simulink model "example_frequency_response"  (R2021b)
settings: Solver=FixedStepDiscrete  StartTime=0.0  StopTime=min(2*3600,15/quadruple_example_frequency_response_f)  FixedStep=0.5  RelTol=1e-3
undefined symbols (not defined in the file or in its folder): cte, quadruple_example_frequency_response_A, quadruple_example_frequency_response_Ai, quadruple_example_frequency_response_f
libraries: sldrtlib x1, simulink x1
settings Model: Creator=IST  LastModifiedBy=IST

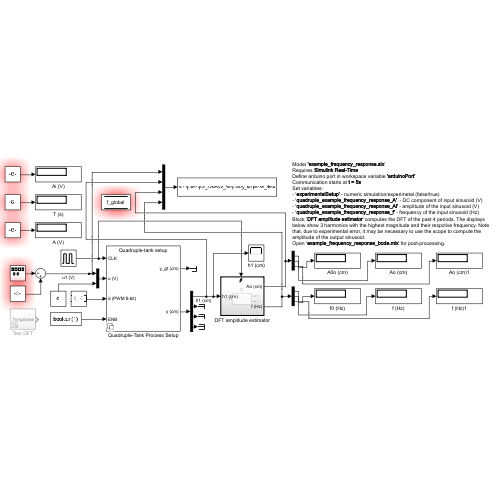
[thumbnail: Simulink's stored preview of the top-level diagram]
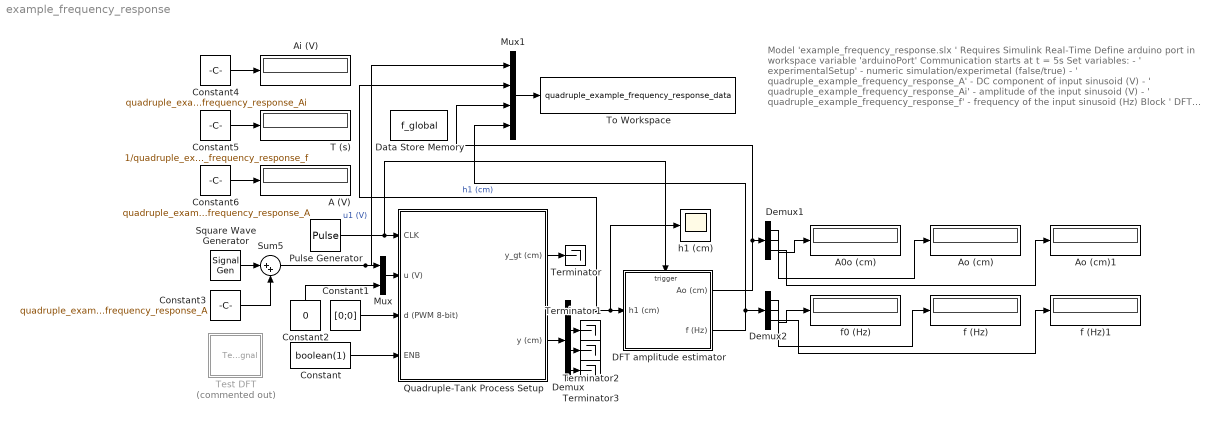
== system example_frequency_response ==
  note: Model 'example_frequency_response.slx '
      | Requires Simulink Real-Time
      | Define arduino port in workspace variable 'arduinoPort'
      | Communication starts at t = 5s
      | Set variables:
      | - ' experimentalSetup' - numeric simulation/experimetal (false/true)
      | - ' quadruple_example_frequency_response_A' - DC component of input sinusoid (V)
      | - ' quadruple_example_frequency_response_Ai' - amplitude of the input sinusoid (V)
      | - ' quadruple_example_frequency_response_f' - frequency of the input sinusoid (Hz)
      | Block ' DFT amplitude estimator ' computes the DFT of the past 4 periods. The displays below show 3 harmonics with the highest magnitude and their respctive frequency. Note that, due to experimental error, it may be necessary to use the scope to compute the amplitude of the output sinusoid.
      | Open ' example_frequency_response_bode.mlx ' for post-processing.
  A (V) : Display
  A0o (cm) : Display
  Ai (V) : Display
  Ao (cm) : Display
  Ao (cm)1 : Display
  Constant : Constant  Priority=4  Value=boolean(1)
  Constant1 : Constant  Value=[0;0]
  Constant2 : Constant  Value=0
  Constant3 : Constant  Value=quadruple_example_frequency_response_A
  Constant4 : Constant  Value=quadruple_example_frequency_response_Ai
  Constant5 : Constant  Value=1/quadruple_example_frequency_response_f
  Constant6 : Constant  Value=quadruple_example_frequency_response_A
  DFT amplitude estimator : Subsystem
  Data Store Memory : DataStoreMemory  DataStoreName=f_global  ReadBeforeWriteMsg=warning  WriteAfterWriteMsg=warning  WriteAfterReadMsg=warning  InitialValue=quadruple_example_frequency_response_f  ShowAdditionalParam=off  OutDataTypeStr=double
  Demux : Demux
  Demux1 : Demux  Outputs=3
  Demux2 : Demux  Outputs=3
  Mux : Mux  Inputs=2
  Mux1 : Mux
  Pulse Generator : DiscretePulseGenerator  PulseType=Time based  Period=1  PulseWidth=50
  Quadruple-Tank Process Setup : Subsystem  InitFcn=|  StopFcn=|  Variant=on
      InitFcn=|
      | % Load parameters
      | cte = quadrupleLoadParameters();
      | % Select simulation mode if unspecified
      | if ~exist('experimentalSetup')
      | experimentalSetup = false;
      | end
      | if experimentalSetup
      | if exist('arduinoPort')
      | if ~isempty(instrfind)
      | fclose(instrfind);
      | delete(instrfind);
      | end
      | arduino = serial(arduinoPort,...
      |                 'BaudRate',9600,...
      |                 'ByteOrder','bigEndian',...
      |                 'DataBits',8,...
      |                 'StopBits',1,...
      |                 'Terminator','');
      | arduino.Parity = 'none';
      | fopen(arduino);
      | else
      | error("Error: Arduino port undefined. Define the port in workspace variable 'arduinoPort'.");
      | end
      | end
      StopFcn=|
      | if experimentalSetup
      | fclose(arduino);
      | end
  Square Wave Generator : SignalGenerator  Amplitude=quadruple_example_frequency_response_Ai  Frequency=quadruple_example_frequency_response_f
  Sum5 : Sum  Inputs=|++
  T (s) : Display
  Terminator{,1..3} (4 alike) : Terminator
  Test DFT : Subsystem  Commented=on
  To Workspace : ToWorkspace  VariableName=quadruple_example_frequency_response_data  SaveFormat=Timeseries  SampleTime=1
  f (Hz) : Display
  f (Hz)1 : Display
  f0 (Hz) : Display
  h1 (cm) : Scope
  wires:
  Demux1/3 -> Ao (cm)1/1
  Demux1/2 -> Ao (cm)/1
  Demux2/3 -> f (Hz)1/1
  Demux/2 -> Terminator1/1
  Constant5/1 -> T (s)/1
  Demux2/2 -> f (Hz)/1
  DFT amplitude estimator/2(f (Hz)) -> Mux1/4, Demux2/1
  Mux/1 -> Quadruple-Tank Process Setup/2(u (V))
  Demux1/1 -> A0o (cm)/1
  Pulse Generator/1 -> Quadruple-Tank Process Setup/1(CLK), DFT amplitude estimator/Trigger
  Constant6/1 -> A (V)/1
  Constant1/1 -> Quadruple-Tank Process Setup/3(d (PWM 8-bit))
  Constant4/1 -> Ai (V)/1
  Mux1/1 -> To Workspace/1
  Demux2/1 -> f0 (Hz)/1
  DFT amplitude estimator/1(Ao (cm)) -> Demux1/1, Mux1/3
  Square Wave Generator/1 -> Sum5/1
  Sum5/1 -> Mux1/1, Mux/1  "u1 (V)"
  Demux/1 -> Mux1/2, h1 (cm)/1, DFT amplitude estimator/1(h1 (cm))  "h1 (cm)"
  Quadruple-Tank Process Setup/1(y_gt (cm)) -> Terminator/1
  Constant3/1 -> Sum5/2
  Quadruple-Tank Process Setup/2(y (cm)) -> Demux/1
  Constant2/1 -> Mux/2
  Demux/3 -> Terminator2/1
  Demux/4 -> Terminator3/1
  Constant/1 -> Quadruple-Tank Process Setup/4(ENB)

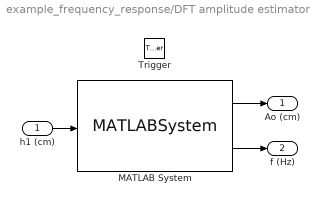
== system example_frequency_response/DFT amplitude estimator ==
  h1 (cm) : Inport
  Trigger : TriggerPort  VariantControl=Variant  PortDimensions=1
  MATLAB System : MATLABSystem  System=output_amplitude_dft  SimulateUsing=Code generation
      mask Type: output_amplitude_dft
      mask Display:
      | disp('output_amplitude_dft');
      | port_label('input',1,'y');
      | port_label('output',1,'Ao');
      | port_label('output',2,'f');
  Ao (cm) : Outport  VectorParamsAs1DForOutWhenUnconnected=off
  f (Hz) : Outport  Port=2  VectorParamsAs1DForOutWhenUnconnected=off
  wires:
  MATLAB System/1 -> Ao (cm)/1
  h1 (cm)/1 -> MATLAB System/1
  MATLAB System/2 -> f (Hz)/1

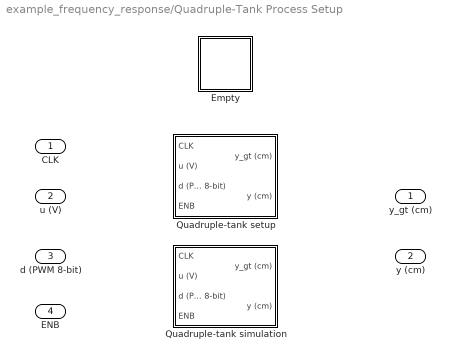
== system example_frequency_response/Quadruple-Tank Process Setup ==
  CLK : Inport
  u (V) : Inport  Port=2
  d (PWM 8-bit) : Inport  Port=3
  ENB : Inport  Port=4
  Empty : Subsystem  VariantControl=%
  Quadruple-tank setup : Subsystem  VariantControl=experimentalSetup == true
  Quadruple-tank simulation : Subsystem  Priority=4  VariantControl=experimentalSetup == false
  y_gt (cm) : Outport  VectorParamsAs1DForOutWhenUnconnected=off
  y (cm) : Outport  Port=2  VectorParamsAs1DForOutWhenUnconnected=off

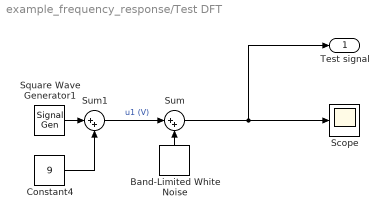
== system example_frequency_response/Test DFT ==
  Band-Limited White Noise : simulink/Sources/Band-Limited White Noise  Cov=0.001  Ts=1  seed=[23341]
  Constant4 : Constant  Value=9
  Scope : Scope
  Square Wave Generator1 : SignalGenerator  Amplitude=quadruple_example_frequency_response_Ai  Frequency=quadruple_example_frequency_response_f
  Sum : Sum  Inputs=|++
  Sum1 : Sum  Inputs=|++
  Test signal : Outport  VectorParamsAs1DForOutWhenUnconnected=off
  wires:
  Sum1/1 -> Sum/1  "u1 (V)"
  Square Wave Generator1/1 -> Sum1/1
  Band-Limited White Noise/1 -> Sum/2
  Constant4/1 -> Sum1/2
  Sum/1 -> Test signal/1, Scope/1

== system example_frequency_response/Quadruple-Tank Process Setup/Empty ==

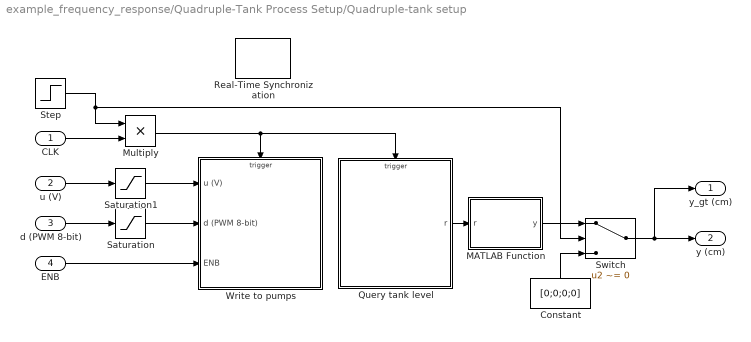
== system example_frequency_response/Quadruple-Tank Process Setup/Quadruple-tank setup ==
  CLK : Inport
  u (V) : Inport  Port=2
  d (PWM 8-bit) : Inport  Port=3
  ENB : Inport  Port=4
  Constant : Constant  Value=[0;0;0;0]
  MATLAB Function : MATLAB Function  TreatAsAtomicUnit=on
  Multiply : Product
  Query tank level : Subsystem  Priority=1
  Real-Time Synchronization : sldrtlib/Real-Time Synchronization  Priority=5  SampleTime=0.5  MaxMissedTicks=10  ShowMissedTicks=off  YieldWhenWaiting=off
  Saturation : Saturate  UpperLimit=255  LowerLimit=0
  Saturation1 : Saturate  UpperLimit=cte.uMax  LowerLimit=cte.uMin
  Step : Step  Time=5  SampleTime=0
  Switch : Switch  Criteria=u2 ~= 0
  Write to pumps : Subsystem  Priority=100
  y_gt (cm) : Outport  VectorParamsAs1DForOutWhenUnconnected=off
  y (cm) : Outport  Port=2  VectorParamsAs1DForOutWhenUnconnected=off
  wires:
  ENB/1 -> Write to pumps/3(ENB)
  Query tank level/1(r) -> MATLAB Function/1(r)
  d (PWM 8-bit)/1 -> Saturation/1
  Saturation/1 -> Write to pumps/2(d (PWM 8-bit))
  u (V)/1 -> Saturation1/1
  Saturation1/1 -> Write to pumps/1(u (V))
  MATLAB Function/1(y) -> Switch/1
  Switch/1 -> y_gt (cm)/1, y (cm)/1
  Constant/1 -> Switch/3
  Step/1 -> Multiply/1, Switch/2
  CLK/1 -> Multiply/2
  Multiply/1 -> Write to pumps/Trigger, Query tank level/Trigger

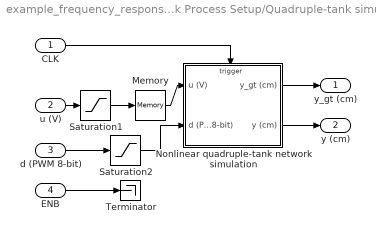
== system example_frequency_response/Quadruple-Tank Process Setup/Quadruple-tank simulation ==
  CLK : Inport
  u (V) : Inport  Port=2
  d (PWM 8-bit) : Inport  Port=3
  ENB : Inport  Port=4
  Memory : Memory
  Nonlinear quadruple-tank network simulation : Subsystem  Priority=10
  Saturation1 : Saturate  UpperLimit=cte.uMax  LowerLimit=cte.uMin
  Saturation2 : Saturate  UpperLimit=2^8-1  LowerLimit=0
  Terminator : Terminator
  y_gt (cm) : Outport  VectorParamsAs1DForOutWhenUnconnected=off
  y (cm) : Outport  Port=2  VectorParamsAs1DForOutWhenUnconnected=off
  wires:
  CLK/1 -> Nonlinear quadruple-tank network simulation/Trigger
  Nonlinear quadruple-tank network simulation/2(y (cm)) -> y (cm)/1
  ENB/1 -> Terminator/1
  Memory/1 -> Nonlinear quadruple-tank network simulation/1(u (V))
  Nonlinear quadruple-tank network simulation/1(y_gt (cm)) -> y_gt (cm)/1
  d (PWM 8-bit)/1 -> Saturation2/1
  u (V)/1 -> Saturation1/1
  Saturation1/1 -> Memory/1
  Saturation2/1 -> Nonlinear quadruple-tank network simulation/2(d (PWM 8-bit))

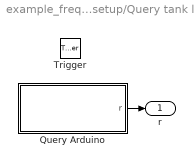
== system example_frequency_response/Quadruple-Tank Process Setup/Quadruple-tank setup/Query tank level ==
  Trigger : TriggerPort  VariantControl=Variant  PortDimensions=1
  Query Arduino : MATLAB Function  TreatAsAtomicUnit=on
  r : Outport  VectorParamsAs1DForOutWhenUnconnected=off
  wires:
  Query Arduino/1(r) -> r/1

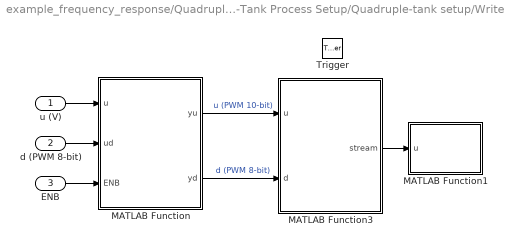
== system example_frequency_response/Quadruple-Tank Process Setup/Quadruple-tank setup/Write to pumps ==
  u (V) : Inport
  d (PWM 8-bit) : Inport  Port=2
  ENB : Inport  Port=3
  Trigger : TriggerPort  VariantControl=Variant  PortDimensions=1
  MATLAB Function : MATLAB Function  TreatAsAtomicUnit=on
  MATLAB Function1 : MATLAB Function  TreatAsAtomicUnit=on
  MATLAB Function3 : MATLAB Function  TreatAsAtomicUnit=on
  wires:
  MATLAB Function/1(yu) -> MATLAB Function3/1(u)  "u (PWM 10-bit)"
  MATLAB Function/2(yd) -> MATLAB Function3/2(d)  "d (PWM 8-bit)"
  u (V)/1 -> MATLAB Function/1(u)
  d (PWM 8-bit)/1 -> MATLAB Function/2(ud)
  ENB/1 -> MATLAB Function/3(ENB)
  MATLAB Function3/1(stream) -> MATLAB Function1/1(u)

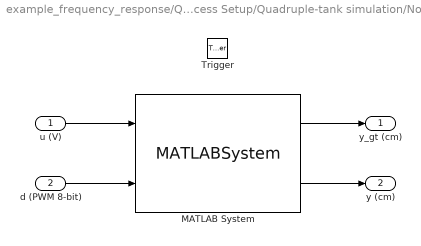
== system example_frequency_response/Quadruple-Tank Process Setup/Quadruple-tank simulation/Nonlinear quadruple-tank network simulation ==
  u (V) : Inport
  d (PWM 8-bit) : Inport  Port=2
  Trigger : TriggerPort  VariantControl=Variant  PortDimensions=1
  MATLAB System : MATLABSystem  System=quadrupleSimObj  SimulateUsing=Interpreted execution
      mask Type: quadrupleSimObj
      mask Display:
      | disp('quadrupleSimObj');
      | port_label('input',1,'u');
      | port_label('input',2,'d');
      | port_label('output',1,'y_gt');
      | port_label('output',2,'y');
  y_gt (cm) : Outport  VectorParamsAs1DForOutWhenUnconnected=off
  y (cm) : Outport  Port=2  VectorParamsAs1DForOutWhenUnconnected=off
  wires:
  u (V)/1 -> MATLAB System/1
  MATLAB System/1 -> y_gt (cm)/1
  MATLAB System/2 -> y (cm)/1
  d (PWM 8-bit)/1 -> MATLAB System/2

== matlab function example_frequency_response/Quadruple-Tank Process Setup/Quadruple-tank setup/Write to pumps/MATLAB Function1 ==
  data: u input
function toArduino(u)
% Find arduino serial object
coder.extrinsic('instrfind'); 
persistent arduino;
if isempty(arduino)
    arduino = instrfind('Status','open','Baud',9600);
end
% Send metadata
fprintf(arduino, "#16");
% Send actuation inputs
fwrite(arduino,u,'uint16');
end

== matlab function example_frequency_response/Quadruple-Tank Process Setup/Quadruple-tank setup/Query tank level/Query Arduino ==
  data: r output
function r = queryArduino()
% Find arduino serial object
coder.extrinsic('instrfind'); 
persistent arduino;
if isempty(arduino)
    arduino = instrfind('Status','open','Baud',9600);
end

% Query arduino
fprintf(arduino, '$');
% Ignore metadata
fread(arduino,[4 1],'uint8');
% Read water-level data
aux = fread(arduino,[5 1],'uint16');
u = zeros(5,1);
u(5) = double(aux(5,1));
for i = 1:4
    u(i) = double(aux(i,1));
    u(i) = (u(5)-u(i))/u(i);
end
r = u(1:4);
end

== matlab function example_frequency_response/Quadruple-Tank Process Setup/Quadruple-tank setup/Write to pumps/MATLAB Function ==
  data: u input; ud input; ENB input; yu output; cte parameter; yd output
function [yu,yd] = pwm_u(u,ud,ENB,cte)
% In u in volts
if ENB
    for i = 1:2
        u(i) = 1023*(cte.c(1,i)*cte.c(3,i)-cte.c(2,i)*cte.k(i)*u(i))/(cte.c(1,i)-cte.k(i)*u(i));
    end
    yu = u;
    yd = ud;
else
    yu = zeros(2,1);
    yd = zeros(2,1);
end

== matlab function example_frequency_response/Quadruple-Tank Process Setup/Quadruple-tank setup/MATLAB Function ==
  data: r input; y output; cte parameter
function y = water_level(r,cte)
y = zeros(4,1);
for i = 1:4
   y(i) = r(i)*cte.dh_dr(i)+cte.h0(i);
end

== matlab function example_frequency_response/Quadruple-Tank Process Setup/Quadruple-tank setup/Write to pumps/MATLAB Function3 ==
  data: u input; stream output; d input
function stream = packPWM10bit(u,d)
    %% Saturation 
    u(u<0) = 0;
    u(u>2^10-1) =2^10-1;
    d(d<0) = 0;
    d(d>2^8-1) =2^8-1;
    %% Pack PWM 
    stream = uint16(zeros(3,1));
    % First two actuation pump signals of 10 bits are sent individually
    stream(1:2) = uint16(round(u)); 
    % Two disturbance pump signals of 8 bits are sent together as a 16 bit
    % uint16_t
    stream(3) = uint16(round(d(1))*2^8+round(d(2)));
end
